simulink model "Lab1"  (R2025b)
settings: Solver=VariableStepAuto  StartTime=0.0  StopTime=0.35  RelTol=1e-3
model workspace (MAT data in the model file):
  J = 3.2284e-06
  K = 0.0274
  Kd = 8e-05
  Ki = 11
  Kp = 0.45
  L = 2.75e-06
  R = 4
  b = 3.5007e-06
settings Model: Creator=jihaoran  LastModifiedBy=jihaoran

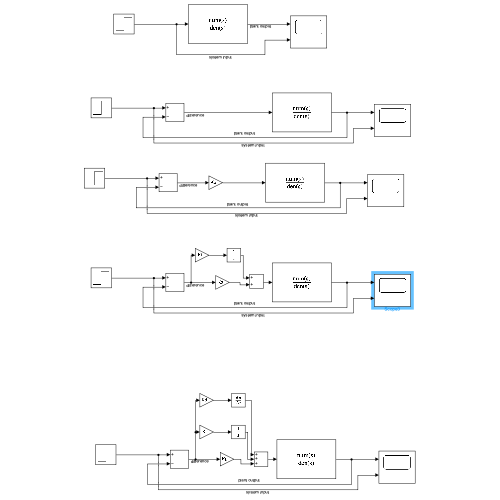
[thumbnail: Simulink's stored preview of the top-level diagram]
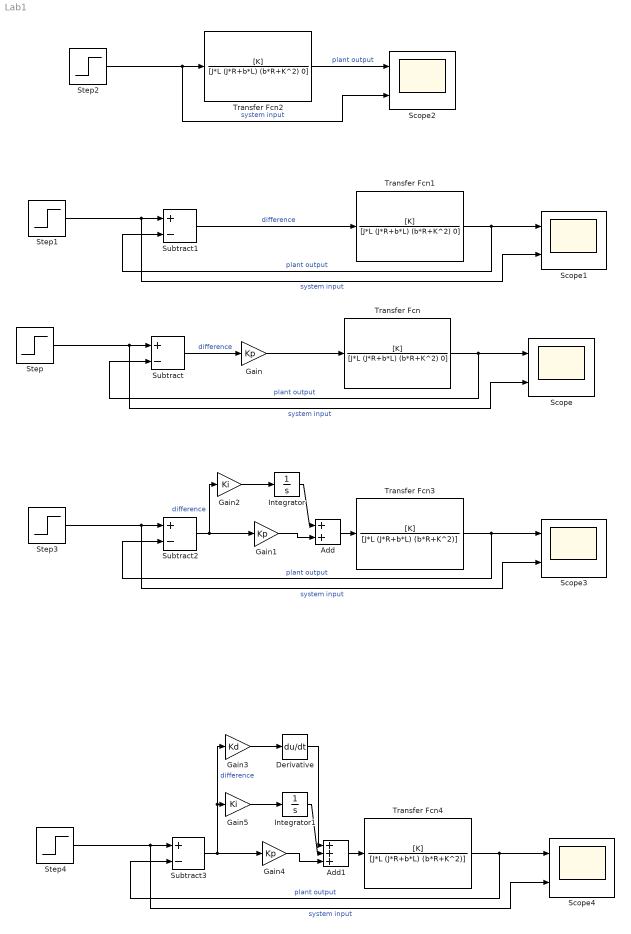
== system Lab1 ==
  Add : Sum
  Add1 : Sum  Inputs=+++
  Derivative : Derivative  CoefficientInTFapproximation=1e-3
  Gain : Gain  Gain=Kp
  Gain1 : Gain  Gain=Kp
  Gain2 : Gain  Gain=Ki
  Gain3 : Gain  Gain=Kd
  Gain4 : Gain  Gain=Kp
  Gain5 : Gain  Gain=Ki
  Integrator : Integrator
  Integrator1 : Integrator
  Scope{,1..4} (5 alike) : Scope  NumInputPorts=2
      Scope settings: ActiveDisplayYMinimum=41.416140114757205  ActiveDisplayYMaximum=71.266941284061019
      Scope1 settings: ActiveDisplayYMinimum=-286.98539398161938  ActiveDisplayYMaximum=166.81091716906874
      Scope2 settings: ActiveDisplayYMinimum=-286.98539398161938  ActiveDisplayYMaximum=166.81091716906874  DataLoggingVariableName=ScopeData2
      Scope3 settings: ActiveDisplayYMinimum=59.706628872191452  ActiveDisplayYMaximum=60.137608408756  DataLoggingVariableName=ScopeData3
      Scope4 settings: ActiveDisplayYMinimum=38.16735276885931  ActiveDisplayYMaximum=67.901128563875233  DataLoggingVariableName=ScopeData4
  Step : Step  Time=0.02  After=60  SampleTime=0
  Step1 : Step  Time=0.02  After=60  SampleTime=0
  Step2 : Step  Time=0.02  After=60  SampleTime=0
  Step3 : Step  Time=0.01  After=60  SampleTime=0
  Step4 : Step  Time=0.01  After=60  SampleTime=0
  Subtract{,1..3} (4 alike) : Sum  Inputs=+-
  Transfer Fcn : TransferFcn  Numerator=[K]  Denominator=[J*L (J*R+b*L) (b*R+K^2) 0]
  Transfer Fcn1 : TransferFcn  Numerator=[K]  Denominator=[J*L (J*R+b*L) (b*R+K^2) 0]
  Transfer Fcn2 : TransferFcn  Numerator=[K]  Denominator=[J*L (J*R+b*L) (b*R+K^2) 0]
  Transfer Fcn3 : TransferFcn  Numerator=[K]  Denominator=[J*L (J*R+b*L) (b*R+K^2)]
  Transfer Fcn4 : TransferFcn  Numerator=[K]  Denominator=[J*L (J*R+b*L) (b*R+K^2)]
  wires:
  Transfer Fcn/1 -> Subtract/2, Scope/1  "plant output"
  Step/1 -> Scope/2, Subtract/1  "system input"
  Subtract/1 -> Gain/1  "difference"
  Gain/1 -> Transfer Fcn/1
  Step1/1 -> Scope1/2, Subtract1/1  "system input"
  Transfer Fcn1/1 -> Subtract1/2, Scope1/1  "plant output"
  Subtract1/1 -> Transfer Fcn1/1  "difference"
  Step2/1 -> Transfer Fcn2/1, Scope2/2  "system input"
  Transfer Fcn2/1 -> Scope2/1  "plant output"
  Step3/1 -> Scope3/2, Subtract2/1  "system input"
  Transfer Fcn3/1 -> Subtract2/2, Scope3/1  "plant output"
  Subtract2/1 -> Gain2/1, Gain1/1  "difference"
  Gain2/1 -> Integrator/1
  Add/1 -> Transfer Fcn3/1
  Gain1/1 -> Add/2
  Integrator/1 -> Add/1
  Add1/1 -> Transfer Fcn4/1
  Integrator1/1 -> Add1/2
  Gain4/1 -> Add1/3
  Step4/1 -> Scope4/2, Subtract3/1  "system input"
  Subtract3/1 -> Gain3/1, Gain5/1, Gain4/1  "difference"
  Transfer Fcn4/1 -> Subtract3/2, Scope4/1  "plant output"
  Gain5/1 -> Integrator1/1
  Gain3/1 -> Derivative/1
  Derivative/1 -> Add1/1
